simulink model "f1"  (R2018b)
settings: Solver=VariableStepAuto  StartTime=0.0  StopTime=10.0  RelTol=1e-3
libraries: fuzblock x1
settings Model: Creator=57035  LastModifiedBy=57035

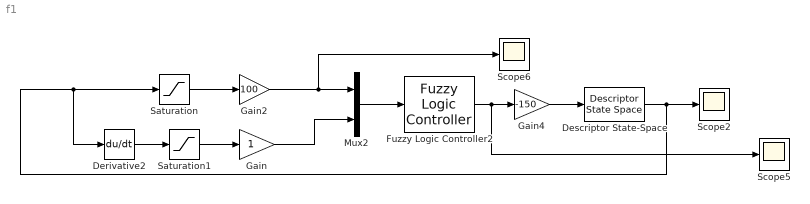
== system f1 ==
  Derivative2 : Derivative
  Descriptor State-Space : DescriptorStateSpace  E=[1,0;0,1]  A=[0,1;38.18,0]  B=[0;-0.195]  C=[1,0]  D=0  InitialCondition=0.1
  Fuzzy Logic Controller2 : fuzblock/Fuzzy Logic  Controller  FIS=e15  OutputSampleNumber=101  DataType=double  FuzzifiedInputs=off  RuleFiringStrengths=off  RuleOutputs=off  AggregatedOutputs=off  SimulateUsing=Interpreted execution  OutOfRangeInputValueMessage=warning  NoRuleFiredMessage=warning  EmptyOutputFuzzySetMessage=warning
  Gain : Gain
  Gain2 : Gain  Gain=100
  Gain4 : Gain  Gain=-150
  Mux2 : Mux  Inputs=2
  Saturation : Saturate
  Saturation1 : Saturate
  Scope2 : Scope
  Scope5 : Scope
  Scope6 : Scope
  wires:
  Saturation1/1 -> Gain/1
  Gain4/1 -> Descriptor State-Space/1
  Mux2/1 -> Fuzzy Logic Controller2/1
  Fuzzy Logic Controller2/1 -> Scope5/1, Gain4/1
  Derivative2/1 -> Saturation1/1
  Descriptor State-Space/1 -> Saturation/1, Derivative2/1, Scope2/1
  Saturation/1 -> Gain2/1
  Gain/1 -> Mux2/2
  Gain2/1 -> Scope6/1, Mux2/1
